simulink model "pfb_fir_generic_test_sim4"  (R2012b)
settings: Solver=VariableStepDiscrete  StartTime=0.0  StopTime=10.0  RelTol=1e-3
model workspace (MAT data in the model file):
  synci = [0 1 2 3 4 5 6 7 8 9 10 11 ... (589826 elements, 294913x2)]
  din0 = [0 1 2 3 4 5 6 7 8 9 10 11 ... (73730 elements, 36865x2)]
  din1 = [0 1 2 3 4 5 6 7 8 9 10 11 ... (73730 elements, 36865x2)]
  din2 = [0 1 2 3 4 5 6 7 8 9 10 11 ... (73730 elements, 36865x2)]
  din3 = [0 1 2 3 4 5 6 7 8 9 10 11 ... (73730 elements, 36865x2)]
  din4 = [0 1 2 3 4 5 6 7 8 9 10 11 ... (73730 elements, 36865x2)]
  din5 = [0 1 2 3 4 5 6 7 8 9 10 11 ... (73730 elements, 36865x2)]
  din6 = [0 1 2 3 4 5 6 7 8 9 10 11 ... (73730 elements, 36865x2)]
  din7 = [0 1 2 3 4 5 6 7 8 9 10 11 ... (73730 elements, 36865x2)]
libraries: xbsIndex_r4 x5323, casper_library_delays x1
(part 9 of 23)

== system pfb_fir_generic_test_sim4/pfb_fir_generic/pfb_fir_coeff_gen/b_expand ==
  bus_in : Inport
  gatewayOut{1..16} (16 alike) : xbsIndex_r4/Gateway Out  inherit_from_input=off  hdl_port=off  timing_constraint=None  locs_specified=off  LOCs={}  UseAsDAC=off  DACChannel='1'  block_type=gatewayout
  reinterpret{1..16} (16 alike) : xbsIndex_r4/Reinterpret  force_arith_type=on  arith_type=Unsigned  force_bin_pt=on  bin_pt=0  block_type=reinterpret
  slice1 : xbsIndex_r4/Slice  nbits=18  boolean_output=off  mode=Upper Bit Location + Width  bit1=-270  base1=MSB of Input  bit0=0  base0=LSB of Input  dbl_ovrd=off  block_type=slice
  slice10 : xbsIndex_r4/Slice  nbits=18  boolean_output=off  mode=Upper Bit Location + Width  bit1=-108  base1=MSB of Input  bit0=0  base0=LSB of Input  dbl_ovrd=off  block_type=slice
  slice11 : xbsIndex_r4/Slice  nbits=18  boolean_output=off  mode=Upper Bit Location + Width  bit1=-90  base1=MSB of Input  bit0=0  base0=LSB of Input  dbl_ovrd=off  block_type=slice
  slice12 : xbsIndex_r4/Slice  nbits=18  boolean_output=off  mode=Upper Bit Location + Width  bit1=-72  base1=MSB of Input  bit0=0  base0=LSB of Input  dbl_ovrd=off  block_type=slice
  slice13 : xbsIndex_r4/Slice  nbits=18  boolean_output=off  mode=Upper Bit Location + Width  bit1=-54  base1=MSB of Input  bit0=0  base0=LSB of Input  dbl_ovrd=off  block_type=slice
  slice14 : xbsIndex_r4/Slice  nbits=18  boolean_output=off  mode=Upper Bit Location + Width  bit1=-36  base1=MSB of Input  bit0=0  base0=LSB of Input  dbl_ovrd=off  block_type=slice
  slice15 : xbsIndex_r4/Slice  nbits=18  boolean_output=off  mode=Upper Bit Location + Width  bit1=-18  base1=MSB of Input  bit0=0  base0=LSB of Input  dbl_ovrd=off  block_type=slice
  slice16 : xbsIndex_r4/Slice  nbits=18  boolean_output=off  mode=Upper Bit Location + Width  bit1=0  base1=MSB of Input  bit0=0  base0=LSB of Input  dbl_ovrd=off  block_type=slice
  slice2 : xbsIndex_r4/Slice  nbits=18  boolean_output=off  mode=Upper Bit Location + Width  bit1=-252  base1=MSB of Input  bit0=0  base0=LSB of Input  dbl_ovrd=off  block_type=slice
  slice3 : xbsIndex_r4/Slice  nbits=18  boolean_output=off  mode=Upper Bit Location + Width  bit1=-234  base1=MSB of Input  bit0=0  base0=LSB of Input  dbl_ovrd=off  block_type=slice
  slice4 : xbsIndex_r4/Slice  nbits=18  boolean_output=off  mode=Upper Bit Location + Width  bit1=-216  base1=MSB of Input  bit0=0  base0=LSB of Input  dbl_ovrd=off  block_type=slice
  slice5 : xbsIndex_r4/Slice  nbits=18  boolean_output=off  mode=Upper Bit Location + Width  bit1=-198  base1=MSB of Input  bit0=0  base0=LSB of Input  dbl_ovrd=off  block_type=slice
  slice6 : xbsIndex_r4/Slice  nbits=18  boolean_output=off  mode=Upper Bit Location + Width  bit1=-180  base1=MSB of Input  bit0=0  base0=LSB of Input  dbl_ovrd=off  block_type=slice
  slice7 : xbsIndex_r4/Slice  nbits=18  boolean_output=off  mode=Upper Bit Location + Width  bit1=-162  base1=MSB of Input  bit0=0  base0=LSB of Input  dbl_ovrd=off  block_type=slice
  slice8 : xbsIndex_r4/Slice  nbits=18  boolean_output=off  mode=Upper Bit Location + Width  bit1=-144  base1=MSB of Input  bit0=0  base0=LSB of Input  dbl_ovrd=off  block_type=slice
  slice9 : xbsIndex_r4/Slice  nbits=18  boolean_output=off  mode=Upper Bit Location + Width  bit1=-126  base1=MSB of Input  bit0=0  base0=LSB of Input  dbl_ovrd=off  block_type=slice
  toWorkspace1 : ToWorkspace  VariableName=coeff_gen_b_expand_1  SampleTime=-1  SaveFormat=Structure With Time
  toWorkspace10 : ToWorkspace  VariableName=coeff_gen_b_expand_10  SampleTime=-1  SaveFormat=Structure With Time
  toWorkspace11 : ToWorkspace  VariableName=coeff_gen_b_expand_11  SampleTime=-1  SaveFormat=Structure With Time
  toWorkspace12 : ToWorkspace  VariableName=coeff_gen_b_expand_12  SampleTime=-1  SaveFormat=Structure With Time
  toWorkspace13 : ToWorkspace  VariableName=coeff_gen_b_expand_13  SampleTime=-1  SaveFormat=Structure With Time
  toWorkspace14 : ToWorkspace  VariableName=coeff_gen_b_expand_14  SampleTime=-1  SaveFormat=Structure With Time
  toWorkspace15 : ToWorkspace  VariableName=coeff_gen_b_expand_15  SampleTime=-1  SaveFormat=Structure With Time
  toWorkspace16 : ToWorkspace  VariableName=coeff_gen_b_expand_16  SampleTime=-1  SaveFormat=Structure With Time
  toWorkspace2 : ToWorkspace  VariableName=coeff_gen_b_expand_2  SampleTime=-1  SaveFormat=Structure With Time
  toWorkspace3 : ToWorkspace  VariableName=coeff_gen_b_expand_3  SampleTime=-1  SaveFormat=Structure With Time
  toWorkspace4 : ToWorkspace  VariableName=coeff_gen_b_expand_4  SampleTime=-1  SaveFormat=Structure With Time
  toWorkspace5 : ToWorkspace  VariableName=coeff_gen_b_expand_5  SampleTime=-1  SaveFormat=Structure With Time
  toWorkspace6 : ToWorkspace  VariableName=coeff_gen_b_expand_6  SampleTime=-1  SaveFormat=Structure With Time
  toWorkspace7 : ToWorkspace  VariableName=coeff_gen_b_expand_7  SampleTime=-1  SaveFormat=Structure With Time
  toWorkspace8 : ToWorkspace  VariableName=coeff_gen_b_expand_8  SampleTime=-1  SaveFormat=Structure With Time
  toWorkspace9 : ToWorkspace  VariableName=coeff_gen_b_expand_9  SampleTime=-1  SaveFormat=Structure With Time
  msb_out16 : Outport
  out15 : Outport  Port=2
  out14 : Outport  Port=3
  out13 : Outport  Port=4
  out12 : Outport  Port=5
  out11 : Outport  Port=6
  out10 : Outport  Port=7
  out9 : Outport  Port=8
  out8 : Outport  Port=9
  out7 : Outport  Port=10
  out6 : Outport  Port=11
  out5 : Outport  Port=12
  out4 : Outport  Port=13
  out3 : Outport  Port=14
  out2 : Outport  Port=15
  lsb_out1 : Outport  Port=16
  wires:
  bus_in/1 -> slice16/1, slice15/1, slice14/1, slice13/1, slice12/1, slice11/1, slice10/1, slice9/1, slice8/1, slice7/1, slice6/1, slice5/1, slice4/1, slice3/1, slice2/1, slice1/1
  slice16/1 -> reinterpret16/1
  reinterpret16/1 -> gatewayOut16/1, msb_out16/1
  gatewayOut16/1 -> toWorkspace16/1
  slice15/1 -> reinterpret15/1
  reinterpret15/1 -> gatewayOut15/1, out15/1
  gatewayOut15/1 -> toWorkspace15/1
  slice14/1 -> reinterpret14/1
  reinterpret14/1 -> gatewayOut14/1, out14/1
  gatewayOut14/1 -> toWorkspace14/1
  slice13/1 -> reinterpret13/1
  reinterpret13/1 -> gatewayOut13/1, out13/1
  gatewayOut13/1 -> toWorkspace13/1
  slice12/1 -> reinterpret12/1
  reinterpret12/1 -> gatewayOut12/1, out12/1
  gatewayOut12/1 -> toWorkspace12/1
  slice11/1 -> reinterpret11/1
  reinterpret11/1 -> gatewayOut11/1, out11/1
  gatewayOut11/1 -> toWorkspace11/1
  slice10/1 -> reinterpret10/1
  reinterpret10/1 -> gatewayOut10/1, out10/1
  gatewayOut10/1 -> toWorkspace10/1
  slice9/1 -> reinterpret9/1
  reinterpret9/1 -> gatewayOut9/1, out9/1
  gatewayOut9/1 -> toWorkspace9/1
  slice8/1 -> reinterpret8/1
  reinterpret8/1 -> gatewayOut8/1, out8/1
  gatewayOut8/1 -> toWorkspace8/1
  slice7/1 -> reinterpret7/1
  reinterpret7/1 -> gatewayOut7/1, out7/1
  gatewayOut7/1 -> toWorkspace7/1
  slice6/1 -> reinterpret6/1
  reinterpret6/1 -> gatewayOut6/1, out6/1
  gatewayOut6/1 -> toWorkspace6/1
  slice5/1 -> reinterpret5/1
  reinterpret5/1 -> gatewayOut5/1, out5/1
  gatewayOut5/1 -> toWorkspace5/1
  slice4/1 -> reinterpret4/1
  reinterpret4/1 -> gatewayOut4/1, out4/1
  gatewayOut4/1 -> toWorkspace4/1
  slice3/1 -> reinterpret3/1
  reinterpret3/1 -> gatewayOut3/1, out3/1
  gatewayOut3/1 -> toWorkspace3/1
  slice2/1 -> reinterpret2/1
  reinterpret2/1 -> gatewayOut2/1, out2/1
  gatewayOut2/1 -> toWorkspace2/1
  slice1/1 -> reinterpret1/1
  reinterpret1/1 -> gatewayOut1/1, lsb_out1/1
  gatewayOut1/1 -> toWorkspace1/1

== system pfb_fir_generic_test_sim4/pfb_fir_generic/pfb_fir_coeff_gen/d0 ==
  in : Inport
  en : Inport  Port=2
  delay_ff : xbsIndex_r4/Delay  rst=off  infoeditControl=Selection of Reset will increase slice count due to use of real FFs and instead of SRLs  en=on  latency=1  dbl_ovrd=off  reg_retiming=off  block_type=delay
  delay_sr : xbsIndex_r4/Delay  rst=off  infoeditControl=Selection of Reset will increase slice count due to use of real FFs and instead of SRLs  en=on  latency=5  dbl_ovrd=off  reg_retiming=on  block_type=delay
  out : Outport
  wires:
  in/1 -> delay_ff/1
  en/1 -> delay_ff/2, delay_sr/2
  delay_ff/1 -> delay_sr/1
  delay_sr/1 -> out/1

== system pfb_fir_generic_test_sim4/pfb_fir_generic/pfb_fir_coeff_gen/d1 ==
  in : Inport
  en : Inport  Port=2
  delay_ff : xbsIndex_r4/Delay  rst=off  infoeditControl=Selection of Reset will increase slice count due to use of real FFs and instead of SRLs  en=on  latency=1  dbl_ovrd=off  reg_retiming=off  block_type=delay
  delay_sr : xbsIndex_r4/Delay  rst=off  infoeditControl=Selection of Reset will increase slice count due to use of real FFs and instead of SRLs  en=on  latency=5  dbl_ovrd=off  reg_retiming=on  block_type=delay
  out : Outport
  wires:
  in/1 -> delay_ff/1
  en/1 -> delay_ff/2, delay_sr/2
  delay_ff/1 -> delay_sr/1
  delay_sr/1 -> out/1

== system pfb_fir_generic_test_sim4/pfb_fir_generic/pfb_fir_coeff_gen/d10 ==
  in : Inport
  en : Inport  Port=2
  delay_ff : xbsIndex_r4/Delay  rst=off  infoeditControl=Selection of Reset will increase slice count due to use of real FFs and instead of SRLs  en=on  latency=1  dbl_ovrd=off  reg_retiming=off  block_type=delay
  delay_sr : xbsIndex_r4/Delay  rst=off  infoeditControl=Selection of Reset will increase slice count due to use of real FFs and instead of SRLs  en=on  latency=3  dbl_ovrd=off  reg_retiming=on  block_type=delay
  out : Outport
  wires:
  in/1 -> delay_ff/1
  en/1 -> delay_ff/2, delay_sr/2
  delay_ff/1 -> delay_sr/1
  delay_sr/1 -> out/1

== system pfb_fir_generic_test_sim4/pfb_fir_generic/pfb_fir_coeff_gen/d11 ==
  in : Inport
  en : Inport  Port=2
  delay_ff : xbsIndex_r4/Delay  rst=off  infoeditControl=Selection of Reset will increase slice count due to use of real FFs and instead of SRLs  en=on  latency=1  dbl_ovrd=off  reg_retiming=off  block_type=delay
  delay_sr : xbsIndex_r4/Delay  rst=off  infoeditControl=Selection of Reset will increase slice count due to use of real FFs and instead of SRLs  en=on  latency=3  dbl_ovrd=off  reg_retiming=on  block_type=delay
  out : Outport
  wires:
  in/1 -> delay_ff/1
  en/1 -> delay_ff/2, delay_sr/2
  delay_ff/1 -> delay_sr/1
  delay_sr/1 -> out/1

== system pfb_fir_generic_test_sim4/pfb_fir_generic/pfb_fir_coeff_gen/d12 ==
  in : Inport
  en : Inport  Port=2
  delay_ff : xbsIndex_r4/Delay  rst=off  infoeditControl=Selection of Reset will increase slice count due to use of real FFs and instead of SRLs  en=on  latency=1  dbl_ovrd=off  reg_retiming=off  block_type=delay
  delay_sr : xbsIndex_r4/Delay  rst=off  infoeditControl=Selection of Reset will increase slice count due to use of real FFs and instead of SRLs  en=on  latency=3  dbl_ovrd=off  reg_retiming=on  block_type=delay
  out : Outport
  wires:
  in/1 -> delay_ff/1
  en/1 -> delay_ff/2, delay_sr/2
  delay_ff/1 -> delay_sr/1
  delay_sr/1 -> out/1

== system pfb_fir_generic_test_sim4/pfb_fir_generic/pfb_fir_coeff_gen/d13 ==
  in : Inport
  en : Inport  Port=2
  delay_ff : xbsIndex_r4/Delay  rst=off  infoeditControl=Selection of Reset will increase slice count due to use of real FFs and instead of SRLs  en=on  latency=1  dbl_ovrd=off  reg_retiming=off  block_type=delay
  delay_sr : xbsIndex_r4/Delay  rst=off  infoeditControl=Selection of Reset will increase slice count due to use of real FFs and instead of SRLs  en=on  latency=3  dbl_ovrd=off  reg_retiming=on  block_type=delay
  out : Outport
  wires:
  in/1 -> delay_ff/1
  en/1 -> delay_ff/2, delay_sr/2
  delay_ff/1 -> delay_sr/1
  delay_sr/1 -> out/1

== system pfb_fir_generic_test_sim4/pfb_fir_generic/pfb_fir_coeff_gen/d14 ==
  in : Inport
  en : Inport  Port=2
  delay_ff : xbsIndex_r4/Delay  rst=off  infoeditControl=Selection of Reset will increase slice count due to use of real FFs and instead of SRLs  en=on  latency=1  dbl_ovrd=off  reg_retiming=off  block_type=delay
  delay_sr : xbsIndex_r4/Delay  rst=off  infoeditControl=Selection of Reset will increase slice count due to use of real FFs and instead of SRLs  en=on  latency=3  dbl_ovrd=off  reg_retiming=on  block_type=delay
  out : Outport
  wires:
  in/1 -> delay_ff/1
  en/1 -> delay_ff/2, delay_sr/2
  delay_ff/1 -> delay_sr/1
  delay_sr/1 -> out/1

== system pfb_fir_generic_test_sim4/pfb_fir_generic/pfb_fir_coeff_gen/d15 ==
  in : Inport
  en : Inport  Port=2
  delay_ff : xbsIndex_r4/Delay  rst=off  infoeditControl=Selection of Reset will increase slice count due to use of real FFs and instead of SRLs  en=on  latency=1  dbl_ovrd=off  reg_retiming=off  block_type=delay
  delay_sr : xbsIndex_r4/Delay  rst=off  infoeditControl=Selection of Reset will increase slice count due to use of real FFs and instead of SRLs  en=on  latency=3  dbl_ovrd=off  reg_retiming=on  block_type=delay
  out : Outport
  wires:
  in/1 -> delay_ff/1
  en/1 -> delay_ff/2, delay_sr/2
  delay_ff/1 -> delay_sr/1
  delay_sr/1 -> out/1

== system pfb_fir_generic_test_sim4/pfb_fir_generic/pfb_fir_coeff_gen/d16 ==
  in : Inport
  en : Inport  Port=2
  delay_ff : xbsIndex_r4/Delay  rst=off  infoeditControl=Selection of Reset will increase slice count due to use of real FFs and instead of SRLs  en=on  latency=1  dbl_ovrd=off  reg_retiming=off  block_type=delay
  delay_sr : xbsIndex_r4/Delay  rst=off  infoeditControl=Selection of Reset will increase slice count due to use of real FFs and instead of SRLs  en=on  latency=1  dbl_ovrd=off  reg_retiming=on  block_type=delay
  out : Outport
  wires:
  in/1 -> delay_ff/1
  en/1 -> delay_ff/2, delay_sr/2
  delay_ff/1 -> delay_sr/1
  delay_sr/1 -> out/1

== system pfb_fir_generic_test_sim4/pfb_fir_generic/pfb_fir_coeff_gen/d17 ==
  in : Inport
  en : Inport  Port=2
  delay_ff : xbsIndex_r4/Delay  rst=off  infoeditControl=Selection of Reset will increase slice count due to use of real FFs and instead of SRLs  en=on  latency=1  dbl_ovrd=off  reg_retiming=off  block_type=delay
  delay_sr : xbsIndex_r4/Delay  rst=off  infoeditControl=Selection of Reset will increase slice count due to use of real FFs and instead of SRLs  en=on  latency=1  dbl_ovrd=off  reg_retiming=on  block_type=delay
  out : Outport
  wires:
  in/1 -> delay_ff/1
  en/1 -> delay_ff/2, delay_sr/2
  delay_ff/1 -> delay_sr/1
  delay_sr/1 -> out/1

== system pfb_fir_generic_test_sim4/pfb_fir_generic/pfb_fir_coeff_gen/d18 ==
  in : Inport
  en : Inport  Port=2
  delay_ff : xbsIndex_r4/Delay  rst=off  infoeditControl=Selection of Reset will increase slice count due to use of real FFs and instead of SRLs  en=on  latency=1  dbl_ovrd=off  reg_retiming=off  block_type=delay
  delay_sr : xbsIndex_r4/Delay  rst=off  infoeditControl=Selection of Reset will increase slice count due to use of real FFs and instead of SRLs  en=on  latency=1  dbl_ovrd=off  reg_retiming=on  block_type=delay
  out : Outport
  wires:
  in/1 -> delay_ff/1
  en/1 -> delay_ff/2, delay_sr/2
  delay_ff/1 -> delay_sr/1
  delay_sr/1 -> out/1

== system pfb_fir_generic_test_sim4/pfb_fir_generic/pfb_fir_coeff_gen/d19 ==
  in : Inport
  en : Inport  Port=2
  delay_ff : xbsIndex_r4/Delay  rst=off  infoeditControl=Selection of Reset will increase slice count due to use of real FFs and instead of SRLs  en=on  latency=1  dbl_ovrd=off  reg_retiming=off  block_type=delay
  delay_sr : xbsIndex_r4/Delay  rst=off  infoeditControl=Selection of Reset will increase slice count due to use of real FFs and instead of SRLs  en=on  latency=1  dbl_ovrd=off  reg_retiming=on  block_type=delay
  out : Outport
  wires:
  in/1 -> delay_ff/1
  en/1 -> delay_ff/2, delay_sr/2
  delay_ff/1 -> delay_sr/1
  delay_sr/1 -> out/1

== system pfb_fir_generic_test_sim4/pfb_fir_generic/pfb_fir_coeff_gen/d2 ==
  in : Inport
  en : Inport  Port=2
  delay_ff : xbsIndex_r4/Delay  rst=off  infoeditControl=Selection of Reset will increase slice count due to use of real FFs and instead of SRLs  en=on  latency=1  dbl_ovrd=off  reg_retiming=off  block_type=delay
  delay_sr : xbsIndex_r4/Delay  rst=off  infoeditControl=Selection of Reset will increase slice count due to use of real FFs and instead of SRLs  en=on  latency=5  dbl_ovrd=off  reg_retiming=on  block_type=delay
  out : Outport
  wires:
  in/1 -> delay_ff/1
  en/1 -> delay_ff/2, delay_sr/2
  delay_ff/1 -> delay_sr/1
  delay_sr/1 -> out/1

== system pfb_fir_generic_test_sim4/pfb_fir_generic/pfb_fir_coeff_gen/d20 ==
  in : Inport
  en : Inport  Port=2
  delay_ff : xbsIndex_r4/Delay  rst=off  infoeditControl=Selection of Reset will increase slice count due to use of real FFs and instead of SRLs  en=on  latency=1  dbl_ovrd=off  reg_retiming=off  block_type=delay
  delay_sr : xbsIndex_r4/Delay  rst=off  infoeditControl=Selection of Reset will increase slice count due to use of real FFs and instead of SRLs  en=on  latency=1  dbl_ovrd=off  reg_retiming=on  block_type=delay
  out : Outport
  wires:
  in/1 -> delay_ff/1
  en/1 -> delay_ff/2, delay_sr/2
  delay_ff/1 -> delay_sr/1
  delay_sr/1 -> out/1

== system pfb_fir_generic_test_sim4/pfb_fir_generic/pfb_fir_coeff_gen/d21 ==
  in : Inport
  en : Inport  Port=2
  delay_ff : xbsIndex_r4/Delay  rst=off  infoeditControl=Selection of Reset will increase slice count due to use of real FFs and instead of SRLs  en=on  latency=1  dbl_ovrd=off  reg_retiming=off  block_type=delay
  delay_sr : xbsIndex_r4/Delay  rst=off  infoeditControl=Selection of Reset will increase slice count due to use of real FFs and instead of SRLs  en=on  latency=1  dbl_ovrd=off  reg_retiming=on  block_type=delay
  out : Outport
  wires:
  in/1 -> delay_ff/1
  en/1 -> delay_ff/2, delay_sr/2
  delay_ff/1 -> delay_sr/1
  delay_sr/1 -> out/1

== system pfb_fir_generic_test_sim4/pfb_fir_generic/pfb_fir_coeff_gen/d22 ==
  in : Inport
  en : Inport  Port=2
  delay_ff : xbsIndex_r4/Delay  rst=off  infoeditControl=Selection of Reset will increase slice count due to use of real FFs and instead of SRLs  en=on  latency=1  dbl_ovrd=off  reg_retiming=off  block_type=delay
  delay_sr : xbsIndex_r4/Delay  rst=off  infoeditControl=Selection of Reset will increase slice count due to use of real FFs and instead of SRLs  en=on  latency=1  dbl_ovrd=off  reg_retiming=on  block_type=delay
  out : Outport
  wires:
  in/1 -> delay_ff/1
  en/1 -> delay_ff/2, delay_sr/2
  delay_ff/1 -> delay_sr/1
  delay_sr/1 -> out/1

== system pfb_fir_generic_test_sim4/pfb_fir_generic/pfb_fir_coeff_gen/d23 ==
  in : Inport
  en : Inport  Port=2
  delay_ff : xbsIndex_r4/Delay  rst=off  infoeditControl=Selection of Reset will increase slice count due to use of real FFs and instead of SRLs  en=on  latency=1  dbl_ovrd=off  reg_retiming=off  block_type=delay
  delay_sr : xbsIndex_r4/Delay  rst=off  infoeditControl=Selection of Reset will increase slice count due to use of real FFs and instead of SRLs  en=on  latency=1  dbl_ovrd=off  reg_retiming=on  block_type=delay
  out : Outport
  wires:
  in/1 -> delay_ff/1
  en/1 -> delay_ff/2, delay_sr/2
  delay_ff/1 -> delay_sr/1
  delay_sr/1 -> out/1

== system pfb_fir_generic_test_sim4/pfb_fir_generic/pfb_fir_coeff_gen/d24 ==
  in : Inport
  en : Inport  Port=2
  delay_ff : xbsIndex_r4/Delay  rst=off  infoeditControl=Selection of Reset will increase slice count due to use of real FFs and instead of SRLs  en=on  latency=1  dbl_ovrd=off  reg_retiming=off  block_type=delay
  out : Outport
  wires:
  in/1 -> delay_ff/1
  en/1 -> delay_ff/2
  delay_ff/1 -> out/1

== system pfb_fir_generic_test_sim4/pfb_fir_generic/pfb_fir_coeff_gen/d25 ==
  in : Inport
  out : Outport
  wires:
  in/1 -> out/1

== system pfb_fir_generic_test_sim4/pfb_fir_generic/pfb_fir_coeff_gen/d26 ==
  in : Inport
  out : Outport
  wires:
  in/1 -> out/1

== system pfb_fir_generic_test_sim4/pfb_fir_generic/pfb_fir_coeff_gen/d27 ==
  in : Inport
  out : Outport
  wires:
  in/1 -> out/1

== system pfb_fir_generic_test_sim4/pfb_fir_generic/pfb_fir_coeff_gen/d28 ==
  in : Inport
  out : Outport
  wires:
  in/1 -> out/1

== system pfb_fir_generic_test_sim4/pfb_fir_generic/pfb_fir_coeff_gen/d29 ==
  in : Inport
  out : Outport
  wires:
  in/1 -> out/1

== system pfb_fir_generic_test_sim4/pfb_fir_generic/pfb_fir_coeff_gen/d3 ==
  in : Inport
  en : Inport  Port=2
  delay_ff : xbsIndex_r4/Delay  rst=off  infoeditControl=Selection of Reset will increase slice count due to use of real FFs and instead of SRLs  en=on  latency=1  dbl_ovrd=off  reg_retiming=off  block_type=delay
  delay_sr : xbsIndex_r4/Delay  rst=off  infoeditControl=Selection of Reset will increase slice count due to use of real FFs and instead of SRLs  en=on  latency=5  dbl_ovrd=off  reg_retiming=on  block_type=delay
  out : Outport
  wires:
  in/1 -> delay_ff/1
  en/1 -> delay_ff/2, delay_sr/2
  delay_ff/1 -> delay_sr/1
  delay_sr/1 -> out/1

== system pfb_fir_generic_test_sim4/pfb_fir_generic/pfb_fir_coeff_gen/d30 ==
  in : Inport
  out : Outport
  wires:
  in/1 -> out/1

== system pfb_fir_generic_test_sim4/pfb_fir_generic/pfb_fir_coeff_gen/d31 ==
  in : Inport
  out : Outport
  wires:
  in/1 -> out/1

== system pfb_fir_generic_test_sim4/pfb_fir_generic/pfb_fir_coeff_gen/d4 ==
  in : Inport
  en : Inport  Port=2
  delay_ff : xbsIndex_r4/Delay  rst=off  infoeditControl=Selection of Reset will increase slice count due to use of real FFs and instead of SRLs  en=on  latency=1  dbl_ovrd=off  reg_retiming=off  block_type=delay
  delay_sr : xbsIndex_r4/Delay  rst=off  infoeditControl=Selection of Reset will increase slice count due to use of real FFs and instead of SRLs  en=on  latency=5  dbl_ovrd=off  reg_retiming=on  block_type=delay
  out : Outport
  wires:
  in/1 -> delay_ff/1
  en/1 -> delay_ff/2, delay_sr/2
  delay_ff/1 -> delay_sr/1
  delay_sr/1 -> out/1

== system pfb_fir_generic_test_sim4/pfb_fir_generic/pfb_fir_coeff_gen/d5 ==
  in : Inport
  en : Inport  Port=2
  delay_ff : xbsIndex_r4/Delay  rst=off  infoeditControl=Selection of Reset will increase slice count due to use of real FFs and instead of SRLs  en=on  latency=1  dbl_ovrd=off  reg_retiming=off  block_type=delay
  delay_sr : xbsIndex_r4/Delay  rst=off  infoeditControl=Selection of Reset will increase slice count due to use of real FFs and instead of SRLs  en=on  latency=5  dbl_ovrd=off  reg_retiming=on  block_type=delay
  out : Outport
  wires:
  in/1 -> delay_ff/1
  en/1 -> delay_ff/2, delay_sr/2
  delay_ff/1 -> delay_sr/1
  delay_sr/1 -> out/1

== system pfb_fir_generic_test_sim4/pfb_fir_generic/pfb_fir_coeff_gen/d6 ==
  in : Inport
  en : Inport  Port=2
  delay_ff : xbsIndex_r4/Delay  rst=off  infoeditControl=Selection of Reset will increase slice count due to use of real FFs and instead of SRLs  en=on  latency=1  dbl_ovrd=off  reg_retiming=off  block_type=delay
  delay_sr : xbsIndex_r4/Delay  rst=off  infoeditControl=Selection of Reset will increase slice count due to use of real FFs and instead of SRLs  en=on  latency=5  dbl_ovrd=off  reg_retiming=on  block_type=delay
  out : Outport
  wires:
  in/1 -> delay_ff/1
  en/1 -> delay_ff/2, delay_sr/2
  delay_ff/1 -> delay_sr/1
  delay_sr/1 -> out/1

== system pfb_fir_generic_test_sim4/pfb_fir_generic/pfb_fir_coeff_gen/d7 ==
  in : Inport
  en : Inport  Port=2
  delay_ff : xbsIndex_r4/Delay  rst=off  infoeditControl=Selection of Reset will increase slice count due to use of real FFs and instead of SRLs  en=on  latency=1  dbl_ovrd=off  reg_retiming=off  block_type=delay
  delay_sr : xbsIndex_r4/Delay  rst=off  infoeditControl=Selection of Reset will increase slice count due to use of real FFs and instead of SRLs  en=on  latency=5  dbl_ovrd=off  reg_retiming=on  block_type=delay
  out : Outport
  wires:
  in/1 -> delay_ff/1
  en/1 -> delay_ff/2, delay_sr/2
  delay_ff/1 -> delay_sr/1
  delay_sr/1 -> out/1

== system pfb_fir_generic_test_sim4/pfb_fir_generic/pfb_fir_coeff_gen/d8 ==
  in : Inport
  en : Inport  Port=2
  delay_ff : xbsIndex_r4/Delay  rst=off  infoeditControl=Selection of Reset will increase slice count due to use of real FFs and instead of SRLs  en=on  latency=1  dbl_ovrd=off  reg_retiming=off  block_type=delay
  delay_sr : xbsIndex_r4/Delay  rst=off  infoeditControl=Selection of Reset will increase slice count due to use of real FFs and instead of SRLs  en=on  latency=3  dbl_ovrd=off  reg_retiming=on  block_type=delay
  out : Outport
  wires:
  in/1 -> delay_ff/1
  en/1 -> delay_ff/2, delay_sr/2
  delay_ff/1 -> delay_sr/1
  delay_sr/1 -> out/1

== system pfb_fir_generic_test_sim4/pfb_fir_generic/pfb_fir_coeff_gen/d9 ==
  in : Inport
  en : Inport  Port=2
  delay_ff : xbsIndex_r4/Delay  rst=off  infoeditControl=Selection of Reset will increase slice count due to use of real FFs and instead of SRLs  en=on  latency=1  dbl_ovrd=off  reg_retiming=off  block_type=delay
  delay_sr : xbsIndex_r4/Delay  rst=off  infoeditControl=Selection of Reset will increase slice count due to use of real FFs and instead of SRLs  en=on  latency=3  dbl_ovrd=off  reg_retiming=on  block_type=delay
  out : Outport
  wires:
  in/1 -> delay_ff/1
  en/1 -> delay_ff/2, delay_sr/2
  delay_ff/1 -> delay_sr/1
  delay_sr/1 -> out/1

== system pfb_fir_generic_test_sim4/pfb_fir_generic/pfb_fir_coeff_gen/en_expand ==
  bus_in : Inport
  slice1 : xbsIndex_r4/Slice  nbits=1  boolean_output=on  mode=Upper Bit Location + Width  bit1=-24  base1=MSB of Input  bit0=0  base0=LSB of Input  dbl_ovrd=off  block_type=slice
  slice10 : xbsIndex_r4/Slice  nbits=1  boolean_output=on  mode=Upper Bit Location + Width  bit1=-15  base1=MSB of Input  bit0=0  base0=LSB of Input  dbl_ovrd=off  block_type=slice
  slice11 : xbsIndex_r4/Slice  nbits=1  boolean_output=on  mode=Upper Bit Location + Width  bit1=-14  base1=MSB of Input  bit0=0  base0=LSB of Input  dbl_ovrd=off  block_type=slice
  slice12 : xbsIndex_r4/Slice  nbits=1  boolean_output=on  mode=Upper Bit Location + Width  bit1=-13  base1=MSB of Input  bit0=0  base0=LSB of Input  dbl_ovrd=off  block_type=slice
  slice13 : xbsIndex_r4/Slice  nbits=1  boolean_output=on  mode=Upper Bit Location + Width  bit1=-12  base1=MSB of Input  bit0=0  base0=LSB of Input  dbl_ovrd=off  block_type=slice
  slice14 : xbsIndex_r4/Slice  nbits=1  boolean_output=on  mode=Upper Bit Location + Width  bit1=-11  base1=MSB of Input  bit0=0  base0=LSB of Input  dbl_ovrd=off  block_type=slice
  slice15 : xbsIndex_r4/Slice  nbits=1  boolean_output=on  mode=Upper Bit Location + Width  bit1=-10  base1=MSB of Input  bit0=0  base0=LSB of Input  dbl_ovrd=off  block_type=slice
  slice16 : xbsIndex_r4/Slice  nbits=1  boolean_output=on  mode=Upper Bit Location + Width  bit1=-9  base1=MSB of Input  bit0=0  base0=LSB of Input  dbl_ovrd=off  block_type=slice
  slice17 : xbsIndex_r4/Slice  nbits=1  boolean_output=on  mode=Upper Bit Location + Width  bit1=-8  base1=MSB of Input  bit0=0  base0=LSB of Input  dbl_ovrd=off  block_type=slice
  slice18 : xbsIndex_r4/Slice  nbits=1  boolean_output=on  mode=Upper Bit Location + Width  bit1=-7  base1=MSB of Input  bit0=0  base0=LSB of Input  dbl_ovrd=off  block_type=slice
  slice19 : xbsIndex_r4/Slice  nbits=1  boolean_output=on  mode=Upper Bit Location + Width  bit1=-6  base1=MSB of Input  bit0=0  base0=LSB of Input  dbl_ovrd=off  block_type=slice
  slice2 : xbsIndex_r4/Slice  nbits=1  boolean_output=on  mode=Upper Bit Location + Width  bit1=-23  base1=MSB of Input  bit0=0  base0=LSB of Input  dbl_ovrd=off  block_type=slice
  slice20 : xbsIndex_r4/Slice  nbits=1  boolean_output=on  mode=Upper Bit Location + Width  bit1=-5  base1=MSB of Input  bit0=0  base0=LSB of Input  dbl_ovrd=off  block_type=slice
  slice21 : xbsIndex_r4/Slice  nbits=1  boolean_output=on  mode=Upper Bit Location + Width  bit1=-4  base1=MSB of Input  bit0=0  base0=LSB of Input  dbl_ovrd=off  block_type=slice
  slice22 : xbsIndex_r4/Slice  nbits=1  boolean_output=on  mode=Upper Bit Location + Width  bit1=-3  base1=MSB of Input  bit0=0  base0=LSB of Input  dbl_ovrd=off  block_type=slice
  slice23 : xbsIndex_r4/Slice  nbits=1  boolean_output=on  mode=Upper Bit Location + Width  bit1=-2  base1=MSB of Input  bit0=0  base0=LSB of Input  dbl_ovrd=off  block_type=slice
  slice24 : xbsIndex_r4/Slice  nbits=1  boolean_output=on  mode=Upper Bit Location + Width  bit1=-1  base1=MSB of Input  bit0=0  base0=LSB of Input  dbl_ovrd=off  block_type=slice
  slice25 : xbsIndex_r4/Slice  nbits=1  boolean_output=on  mode=Upper Bit Location + Width  bit1=0  base1=MSB of Input  bit0=0  base0=LSB of Input  dbl_ovrd=off  block_type=slice
  slice3 : xbsIndex_r4/Slice  nbits=1  boolean_output=on  mode=Upper Bit Location + Width  bit1=-22  base1=MSB of Input  bit0=0  base0=LSB of Input  dbl_ovrd=off  block_type=slice
  slice4 : xbsIndex_r4/Slice  nbits=1  boolean_output=on  mode=Upper Bit Location + Width  bit1=-21  base1=MSB of Input  bit0=0  base0=LSB of Input  dbl_ovrd=off  block_type=slice
  slice5 : xbsIndex_r4/Slice  nbits=1  boolean_output=on  mode=Upper Bit Location + Width  bit1=-20  base1=MSB of Input  bit0=0  base0=LSB of Input  dbl_ovrd=off  block_type=slice
  slice6 : xbsIndex_r4/Slice  nbits=1  boolean_output=on  mode=Upper Bit Location + Width  bit1=-19  base1=MSB of Input  bit0=0  base0=LSB of Input  dbl_ovrd=off  block_type=slice
  slice7 : xbsIndex_r4/Slice  nbits=1  boolean_output=on  mode=Upper Bit Location + Width  bit1=-18  base1=MSB of Input  bit0=0  base0=LSB of Input  dbl_ovrd=off  block_type=slice
  slice8 : xbsIndex_r4/Slice  nbits=1  boolean_output=on  mode=Upper Bit Location + Width  bit1=-17  base1=MSB of Input  bit0=0  base0=LSB of Input  dbl_ovrd=off  block_type=slice
  slice9 : xbsIndex_r4/Slice  nbits=1  boolean_output=on  mode=Upper Bit Location + Width  bit1=-16  base1=MSB of Input  bit0=0  base0=LSB of Input  dbl_ovrd=off  block_type=slice
  msb_out25 : Outport
  out24 : Outport  Port=2
  out23 : Outport  Port=3
  out22 : Outport  Port=4
  out21 : Outport  Port=5
  out20 : Outport  Port=6
  out19 : Outport  Port=7
  out18 : Outport  Port=8
  out17 : Outport  Port=9
  out16 : Outport  Port=10
  out15 : Outport  Port=11
  out14 : Outport  Port=12
  out13 : Outport  Port=13
  out12 : Outport  Port=14
  out11 : Outport  Port=15
  out10 : Outport  Port=16
  out9 : Outport  Port=17
  out8 : Outport  Port=18
  out7 : Outport  Port=19
  out6 : Outport  Port=20
  out5 : Outport  Port=21
  out4 : Outport  Port=22
  out3 : Outport  Port=23
  out2 : Outport  Port=24
  lsb_out1 : Outport  Port=25
  wires:
  bus_in/1 -> slice25/1, slice24/1, slice23/1, slice22/1, slice21/1, slice20/1, slice19/1, slice18/1, slice17/1, slice16/1, slice15/1, slice14/1, slice13/1, slice12/1, slice11/1, slice10/1, slice9/1, slice8/1, slice7/1, slice6/1, slice5/1, slice4/1, slice3/1, slice2/1, slice1/1
  slice25/1 -> msb_out25/1
  slice24/1 -> out24/1
  slice23/1 -> out23/1
  slice22/1 -> out22/1
  slice21/1 -> out21/1
  slice20/1 -> out20/1
  slice19/1 -> out19/1
  slice18/1 -> out18/1
  slice17/1 -> out17/1
  slice16/1 -> out16/1
  slice15/1 -> out15/1
  slice14/1 -> out14/1
  slice13/1 -> out13/1
  slice12/1 -> out12/1
  slice11/1 -> out11/1
  slice10/1 -> out10/1
  slice9/1 -> out9/1
  slice8/1 -> out8/1
  slice7/1 -> out7/1
  slice6/1 -> out6/1
  slice5/1 -> out5/1
  slice4/1 -> out4/1
  slice3/1 -> out3/1
  slice2/1 -> out2/1
  slice1/1 -> lsb_out1/1

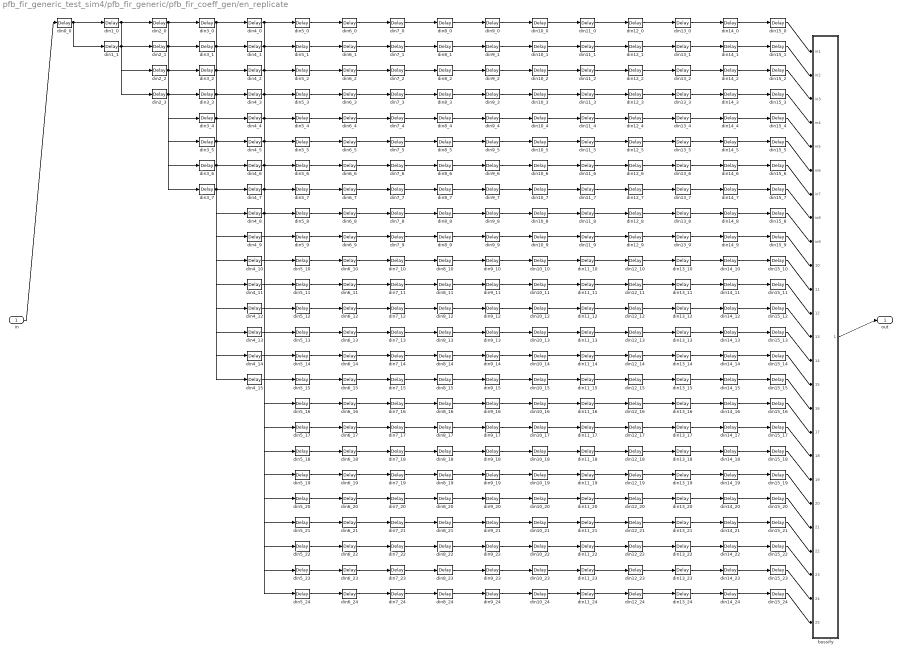
== system pfb_fir_generic_test_sim4/pfb_fir_generic/pfb_fir_coeff_gen/en_replicate ==
  in : Inport
  bussify : Subsystem  AncestorBlock=casper_library_flow_control/bus_create  mask(bus_create){inputNum=25}
      mask prompts: inputNum "Number of inputs:"
      mask init:
      | bus_create_init(gcb,...
      |     'inputNum', inputNum);
  din0_0 : xbsIndex_r4/Delay  rst=off  infoeditControl=Selection of Reset will increase slice count due to use of real FFs and instead of SRLs  en=off  latency=1  dbl_ovrd=off  reg_retiming=off  block_type=delay
  din10_{0..24} (25 alike) : xbsIndex_r4/Delay  rst=off  infoeditControl=Selection of Reset will increase slice count due to use of real FFs and instead of SRLs  en=off  latency=1  dbl_ovrd=off  reg_retiming=on  block_type=delay
  din11_{0..24} (25 alike) : xbsIndex_r4/Delay  rst=off  infoeditControl=Selection of Reset will increase slice count due to use of real FFs and instead of SRLs  en=off  latency=1  dbl_ovrd=off  reg_retiming=on  block_type=delay
  din12_{0..24} (25 alike) : xbsIndex_r4/Delay  rst=off  infoeditControl=Selection of Reset will increase slice count due to use of real FFs and instead of SRLs  en=off  latency=1  dbl_ovrd=off  reg_retiming=on  block_type=delay
  din13_{0..24} (25 alike) : xbsIndex_r4/Delay  rst=off  infoeditControl=Selection of Reset will increase slice count due to use of real FFs and instead of SRLs  en=off  latency=1  dbl_ovrd=off  reg_retiming=on  block_type=delay
  din14_{0..24} (25 alike) : xbsIndex_r4/Delay  rst=off  infoeditControl=Selection of Reset will increase slice count due to use of real FFs and instead of SRLs  en=off  latency=1  dbl_ovrd=off  reg_retiming=on  block_type=delay
  din15_{0..24} (25 alike) : xbsIndex_r4/Delay  rst=off  infoeditControl=Selection of Reset will increase slice count due to use of real FFs and instead of SRLs  en=off  latency=1  dbl_ovrd=off  reg_retiming=off  block_type=delay
  din1_0 : xbsIndex_r4/Delay  rst=off  infoeditControl=Selection of Reset will increase slice count due to use of real FFs and instead of SRLs  en=off  latency=1  dbl_ovrd=off  reg_retiming=off  block_type=delay
  din1_1 : xbsIndex_r4/Delay  rst=off  infoeditControl=Selection of Reset will increase slice count due to use of real FFs and instead of SRLs  en=off  latency=1  dbl_ovrd=off  reg_retiming=off  block_type=delay
  din2_{0..3} (4 alike) : xbsIndex_r4/Delay  rst=off  infoeditControl=Selection of Reset will increase slice count due to use of real FFs and instead of SRLs  en=off  latency=1  dbl_ovrd=off  reg_retiming=off  block_type=delay
  din3_{0..7} (8 alike) : xbsIndex_r4/Delay  rst=off  infoeditControl=Selection of Reset will increase slice count due to use of real FFs and instead of SRLs  en=off  latency=1  dbl_ovrd=off  reg_retiming=off  block_type=delay
  din4_{0..15} (16 alike) : xbsIndex_r4/Delay  rst=off  infoeditControl=Selection of Reset will increase slice count due to use of real FFs and instead of SRLs  en=off  latency=1  dbl_ovrd=off  reg_retiming=off  block_type=delay
  din5_{0..24} (25 alike) : xbsIndex_r4/Delay  rst=off  infoeditControl=Selection of Reset will increase slice count due to use of real FFs and instead of SRLs  en=off  latency=1  dbl_ovrd=off  reg_retiming=on  block_type=delay
  din6_{0..24} (25 alike) : xbsIndex_r4/Delay  rst=off  infoeditControl=Selection of Reset will increase slice count due to use of real FFs and instead of SRLs  en=off  latency=1  dbl_ovrd=off  reg_retiming=on  block_type=delay
  din7_{0..24} (25 alike) : xbsIndex_r4/Delay  rst=off  infoeditControl=Selection of Reset will increase slice count due to use of real FFs and instead of SRLs  en=off  latency=1  dbl_ovrd=off  reg_retiming=on  block_type=delay
  din8_{0..24} (25 alike) : xbsIndex_r4/Delay  rst=off  infoeditControl=Selection of Reset will increase slice count due to use of real FFs and instead of SRLs  en=off  latency=1  dbl_ovrd=off  reg_retiming=on  block_type=delay
  din9_{0..24} (25 alike) : xbsIndex_r4/Delay  rst=off  infoeditControl=Selection of Reset will increase slice count due to use of real FFs and instead of SRLs  en=off  latency=1  dbl_ovrd=off  reg_retiming=on  block_type=delay
  out : Outport
  wires:
  in/1 -> din0_0/1
  din0_0/1 -> din1_0/1, din1_1/1
  din1_0/1 -> din2_0/1, din2_2/1
  din1_1/1 -> din2_1/1, din2_3/1
  din2_0/1 -> din3_0/1, din3_4/1
  din2_1/1 -> din3_1/1, din3_5/1
  din2_2/1 -> din3_2/1, din3_6/1
  din2_3/1 -> din3_3/1, din3_7/1
  din3_0/1 -> din4_0/1, din4_8/1
  din3_1/1 -> din4_1/1, din4_9/1
  din3_2/1 -> din4_2/1, din4_10/1
  din3_3/1 -> din4_3/1, din4_11/1
  din3_4/1 -> din4_4/1, din4_12/1
  din3_5/1 -> din4_5/1, din4_13/1
  din3_6/1 -> din4_6/1, din4_14/1
  din3_7/1 -> din4_7/1, din4_15/1
  din4_0/1 -> din5_0/1, din5_16/1
  din4_1/1 -> din5_1/1, din5_17/1
  din4_2/1 -> din5_2/1, din5_18/1
  din4_3/1 -> din5_3/1, din5_19/1
  din4_4/1 -> din5_4/1, din5_20/1
  din4_5/1 -> din5_5/1, din5_21/1
  din4_6/1 -> din5_6/1, din5_22/1
  din4_7/1 -> din5_7/1, din5_23/1
  din4_8/1 -> din5_8/1, din5_24/1
  din4_9/1 -> din5_9/1
  din4_10/1 -> din5_10/1
  din4_11/1 -> din5_11/1
  din4_12/1 -> din5_12/1
  din4_13/1 -> din5_13/1
  din4_14/1 -> din5_14/1
  din4_15/1 -> din5_15/1
  din5_0/1 -> din6_0/1
  din5_1/1 -> din6_1/1
  din5_2/1 -> din6_2/1
  din5_3/1 -> din6_3/1
  din5_4/1 -> din6_4/1
  din5_5/1 -> din6_5/1
  din5_6/1 -> din6_6/1
  din5_7/1 -> din6_7/1
  din5_8/1 -> din6_8/1
  din5_9/1 -> din6_9/1
  din5_10/1 -> din6_10/1
  din5_11/1 -> din6_11/1
  din5_12/1 -> din6_12/1
  din5_13/1 -> din6_13/1
  din5_14/1 -> din6_14/1
  din5_15/1 -> din6_15/1
  din5_16/1 -> din6_16/1
  din5_17/1 -> din6_17/1
  din5_18/1 -> din6_18/1
  din5_19/1 -> din6_19/1
  din5_20/1 -> din6_20/1
  din5_21/1 -> din6_21/1
  din5_22/1 -> din6_22/1
  din5_23/1 -> din6_23/1
  din5_24/1 -> din6_24/1
  din6_0/1 -> din7_0/1
  din6_1/1 -> din7_1/1
  din6_2/1 -> din7_2/1
  din6_3/1 -> din7_3/1
  din6_4/1 -> din7_4/1
  din6_5/1 -> din7_5/1
  din6_6/1 -> din7_6/1
  din6_7/1 -> din7_7/1
  din6_8/1 -> din7_8/1
  din6_9/1 -> din7_9/1
  din6_10/1 -> din7_10/1
  din6_11/1 -> din7_11/1
  din6_12/1 -> din7_12/1
  din6_13/1 -> din7_13/1
  din6_14/1 -> din7_14/1
  din6_15/1 -> din7_15/1
  din6_16/1 -> din7_16/1
  din6_17/1 -> din7_17/1
  din6_18/1 -> din7_18/1
  din6_19/1 -> din7_19/1
  din6_20/1 -> din7_20/1
  din6_21/1 -> din7_21/1
  din6_22/1 -> din7_22/1
  din6_23/1 -> din7_23/1
  din6_24/1 -> din7_24/1
  din7_0/1 -> din8_0/1
  din7_1/1 -> din8_1/1
  din7_2/1 -> din8_2/1
  din7_3/1 -> din8_3/1
  din7_4/1 -> din8_4/1
  din7_5/1 -> din8_5/1
  din7_6/1 -> din8_6/1
  din7_7/1 -> din8_7/1
  din7_8/1 -> din8_8/1
  din7_9/1 -> din8_9/1
  din7_10/1 -> din8_10/1
  din7_11/1 -> din8_11/1
  din7_12/1 -> din8_12/1
  din7_13/1 -> din8_13/1
  din7_14/1 -> din8_14/1
  din7_15/1 -> din8_15/1
  din7_16/1 -> din8_16/1
  din7_17/1 -> din8_17/1
  din7_18/1 -> din8_18/1
  din7_19/1 -> din8_19/1
  din7_20/1 -> din8_20/1
  din7_21/1 -> din8_21/1
  din7_22/1 -> din8_22/1
  din7_23/1 -> din8_23/1
  din7_24/1 -> din8_24/1
  din8_0/1 -> din9_0/1
  din8_1/1 -> din9_1/1
  din8_2/1 -> din9_2/1
  din8_3/1 -> din9_3/1
  din8_4/1 -> din9_4/1
  din8_5/1 -> din9_5/1
  din8_6/1 -> din9_6/1
  din8_7/1 -> din9_7/1
  din8_8/1 -> din9_8/1
  din8_9/1 -> din9_9/1
  din8_10/1 -> din9_10/1
  din8_11/1 -> din9_11/1
  din8_12/1 -> din9_12/1
  din8_13/1 -> din9_13/1
  din8_14/1 -> din9_14/1
  din8_15/1 -> din9_15/1
  din8_16/1 -> din9_16/1
  din8_17/1 -> din9_17/1
  din8_18/1 -> din9_18/1
  din8_19/1 -> din9_19/1
  din8_20/1 -> din9_20/1
  din8_21/1 -> din9_21/1
  din8_22/1 -> din9_22/1
  din8_23/1 -> din9_23/1
  din8_24/1 -> din9_24/1
  din9_0/1 -> din10_0/1
  din9_1/1 -> din10_1/1
  din9_2/1 -> din10_2/1
  din9_3/1 -> din10_3/1
  din9_4/1 -> din10_4/1
  din9_5/1 -> din10_5/1
  din9_6/1 -> din10_6/1
  din9_7/1 -> din10_7/1
  din9_8/1 -> din10_8/1
  din9_9/1 -> din10_9/1
  din9_10/1 -> din10_10/1
  din9_11/1 -> din10_11/1
  din9_12/1 -> din10_12/1
  din9_13/1 -> din10_13/1
  din9_14/1 -> din10_14/1
  din9_15/1 -> din10_15/1
  din9_16/1 -> din10_16/1
  din9_17/1 -> din10_17/1
  din9_18/1 -> din10_18/1
  din9_19/1 -> din10_19/1
  din9_20/1 -> din10_20/1
  din9_21/1 -> din10_21/1
  din9_22/1 -> din10_22/1
  din9_23/1 -> din10_23/1
  din9_24/1 -> din10_24/1
  din10_0/1 -> din11_0/1
  din10_1/1 -> din11_1/1
  din10_2/1 -> din11_2/1
  din10_3/1 -> din11_3/1
  din10_4/1 -> din11_4/1
  din10_5/1 -> din11_5/1
  din10_6/1 -> din11_6/1
  din10_7/1 -> din11_7/1
  din10_8/1 -> din11_8/1
  din10_9/1 -> din11_9/1
  din10_10/1 -> din11_10/1
  din10_11/1 -> din11_11/1
  din10_12/1 -> din11_12/1
  din10_13/1 -> din11_13/1
  din10_14/1 -> din11_14/1
  din10_15/1 -> din11_15/1
  din10_16/1 -> din11_16/1
  din10_17/1 -> din11_17/1
  din10_18/1 -> din11_18/1
  din10_19/1 -> din11_19/1
  din10_20/1 -> din11_20/1
  din10_21/1 -> din11_21/1
  din10_22/1 -> din11_22/1
  din10_23/1 -> din11_23/1
  din10_24/1 -> din11_24/1
  din11_0/1 -> din12_0/1
  din11_1/1 -> din12_1/1
  din11_2/1 -> din12_2/1
  din11_3/1 -> din12_3/1
  din11_4/1 -> din12_4/1
  din11_5/1 -> din12_5/1
  din11_6/1 -> din12_6/1
  din11_7/1 -> din12_7/1
  din11_8/1 -> din12_8/1
  din11_9/1 -> din12_9/1
  din11_10/1 -> din12_10/1
  din11_11/1 -> din12_11/1
  din11_12/1 -> din12_12/1
  din11_13/1 -> din12_13/1
  din11_14/1 -> din12_14/1
  din11_15/1 -> din12_15/1
  din11_16/1 -> din12_16/1
  din11_17/1 -> din12_17/1
  din11_18/1 -> din12_18/1
  din11_19/1 -> din12_19/1
  din11_20/1 -> din12_20/1
  din11_21/1 -> din12_21/1
  din11_22/1 -> din12_22/1
  din11_23/1 -> din12_23/1
  din11_24/1 -> din12_24/1
  din12_0/1 -> din13_0/1
  din12_1/1 -> din13_1/1
  din12_2/1 -> din13_2/1
  din12_3/1 -> din13_3/1
  din12_4/1 -> din13_4/1
  din12_5/1 -> din13_5/1
  din12_6/1 -> din13_6/1
  din12_7/1 -> din13_7/1
  din12_8/1 -> din13_8/1
  din12_9/1 -> din13_9/1
  din12_10/1 -> din13_10/1
  din12_11/1 -> din13_11/1
  din12_12/1 -> din13_12/1
  din12_13/1 -> din13_13/1
  din12_14/1 -> din13_14/1
  din12_15/1 -> din13_15/1
  din12_16/1 -> din13_16/1
  din12_17/1 -> din13_17/1
  din12_18/1 -> din13_18/1
  din12_19/1 -> din13_19/1
  din12_20/1 -> din13_20/1
  din12_21/1 -> din13_21/1
  din12_22/1 -> din13_22/1
  din12_23/1 -> din13_23/1
  din12_24/1 -> din13_24/1
  din13_0/1 -> din14_0/1
  din13_1/1 -> din14_1/1
  din13_2/1 -> din14_2/1
  din13_3/1 -> din14_3/1
  din13_4/1 -> din14_4/1
  din13_5/1 -> din14_5/1
  din13_6/1 -> din14_6/1
  din13_7/1 -> din14_7/1
  din13_8/1 -> din14_8/1
  din13_9/1 -> din14_9/1
  din13_10/1 -> din14_10/1
  din13_11/1 -> din14_11/1
  din13_12/1 -> din14_12/1
  din13_13/1 -> din14_13/1
  din13_14/1 -> din14_14/1
  din13_15/1 -> din14_15/1
  din13_16/1 -> din14_16/1
  din13_17/1 -> din14_17/1
  din13_18/1 -> din14_18/1
  din13_19/1 -> din14_19/1
  din13_20/1 -> din14_20/1
  din13_21/1 -> din14_21/1
  din13_22/1 -> din14_22/1
  din13_23/1 -> din14_23/1
  din13_24/1 -> din14_24/1
  din14_0/1 -> din15_0/1
  din14_1/1 -> din15_1/1
  din14_2/1 -> din15_2/1
  din14_3/1 -> din15_3/1
  din14_4/1 -> din15_4/1
  din14_5/1 -> din15_5/1
  din14_6/1 -> din15_6/1
  din14_7/1 -> din15_7/1
  din14_8/1 -> din15_8/1
  din14_9/1 -> din15_9/1
  din14_10/1 -> din15_10/1
  din14_11/1 -> din15_11/1
  din14_12/1 -> din15_12/1
  din14_13/1 -> din15_13/1
  din14_14/1 -> din15_14/1
  din14_15/1 -> din15_15/1
  din14_16/1 -> din15_16/1
  din14_17/1 -> din15_17/1
  din14_18/1 -> din15_18/1
  din14_19/1 -> din15_19/1
  din14_20/1 -> din15_20/1
  din14_21/1 -> din15_21/1
  din14_22/1 -> din15_22/1
  din14_23/1 -> din15_23/1
  din14_24/1 -> din15_24/1
  din15_0/1 -> bussify/1(in1)
  din15_1/1 -> bussify/2(in2)
  din15_2/1 -> bussify/3(in3)
  din15_3/1 -> bussify/4(in4)
  din15_4/1 -> bussify/5(in5)
  din15_5/1 -> bussify/6(in6)
  din15_6/1 -> bussify/7(in7)
  din15_7/1 -> bussify/8(in8)
  din15_8/1 -> bussify/9(in9)
  din15_9/1 -> bussify/10(in10)
  din15_10/1 -> bussify/11(in11)
  din15_11/1 -> bussify/12(in12)
  din15_12/1 -> bussify/13(in13)
  din15_13/1 -> bussify/14(in14)
  din15_14/1 -> bussify/15(in15)
  din15_15/1 -> bussify/16(in16)
  din15_16/1 -> bussify/17(in17)
  din15_17/1 -> bussify/18(in18)
  din15_18/1 -> bussify/19(in19)
  din15_19/1 -> bussify/20(in20)
  din15_20/1 -> bussify/21(in21)
  din15_21/1 -> bussify/22(in22)
  din15_22/1 -> bussify/23(in23)
  din15_23/1 -> bussify/24(in24)
  din15_24/1 -> bussify/25(in25)
  bussify/1(bus_out) -> out/1

== system pfb_fir_generic_test_sim4/pfb_fir_generic/pfb_fir_coeff_gen/munge ==
  din : Inport
  join : Subsystem  AncestorBlock=casper_library_flow_control/bus_create  mask(bus_create){inputNum=16}
      mask prompts: inputNum "Number of inputs:"
      mask init:
      | bus_create_init(gcb,...
      |     'inputNum', inputNum);
  reinterpret : xbsIndex_r4/Reinterpret  force_arith_type=on  arith_type=Unsigned  force_bin_pt=on  bin_pt=0  block_type=reinterpret
  reinterpret_out : xbsIndex_r4/Reinterpret  force_arith_type=on  arith_type=Unsigned  force_bin_pt=on  bin_pt=0  block_type=reinterpret
  split : Subsystem  AncestorBlock=casper_library_flow_control/bus_expand  mask(bus_expand){mode=divisions of arbitrary size, outputNum=1, outputWidth=[18 18 18 18 18 18 18 18 18 18 18 18 18 18 18 18], outputBinaryPt=[0 0 0 0 0 0 0 0 0 0 0 0 0 0 0 0], outputArithmeticType=[0 0 0 0 0 0 0 0 0 0 0 0 0 0 0 0], show_format=off, outputToWorkspace=off, variablePrefix=out, outputToModelAsWell=on}
      mask prompts: outputNum "Number of outputs:"; outputWidth "Output width [msb ... lsb]:"; outputBinaryPt "Output binary point position [msb ... lsb]:"; outputArithmeticType "Output arithmetic type (ufix=0, fix=1, bool=2) [msb ... lsb]:"; show_format "Print format string?"; outputToWorkspace "Output to workspace?"; variablePrefix "Variable name prefix:"; outputToModelAsWell "Output to model as well?"
      mask help:
      | Expands a 'bus' made using a bus_create or Xilinx
      | concat block.
      | The input will be divided into the specified number
      | of outputs with the specified arithmetic types.
      | Divisions are made from most significant bit.
      mask init: same as pfb_fir_generic_test_sim4/pfb_fir_generic/bus_expand
      settings: AttributesFormatString=16 outputs
      mask TypeOptions mode: divisions of equal size | divisions of arbitrary size
      mask Callback mode: bus_expand_callback();
      mask Callback outputWidth: bus_expand_callback();
      mask Callback outputToWorkspace: bus_expand_callback();
  dout : Outport
  wires:
  reinterpret_out/1 -> dout/1
  din/1 -> reinterpret/1
  reinterpret/1 -> split/1(bus_in)
  join/1(bus_out) -> reinterpret_out/1
  split/9(out8) -> join/1(in1)
  split/16(lsb_out1) -> join/2(in2)
  split/15(out2) -> join/3(in3)
  split/14(out3) -> join/4(in4)
  split/13(out4) -> join/5(in5)
  split/12(out5) -> join/6(in6)
  split/11(out6) -> join/7(in7)
  split/10(out7) -> join/8(in8)
  split/1(msb_out16) -> join/9(in9)
  split/8(out9) -> join/10(in10)
  split/7(out10) -> join/11(in11)
  split/6(out11) -> join/12(in12)
  split/5(out12) -> join/13(in13)
  split/4(out13) -> join/14(in14)
  split/3(out14) -> join/15(in15)
  split/2(out15) -> join/16(in16)
